simulink model "SCARA_Control_System"  (R2023a)
settings: Solver=VariableStepAuto  StartTime=0.0  StopTime=10.0  RelTol=1e-3
undefined symbols (not defined in the file): X, Y, Z
libraries: sm_lib x25, nesl_utility x16, robotcorelib x1
settings Model: Creator=Memoh  LastModifiedBy=Memoh

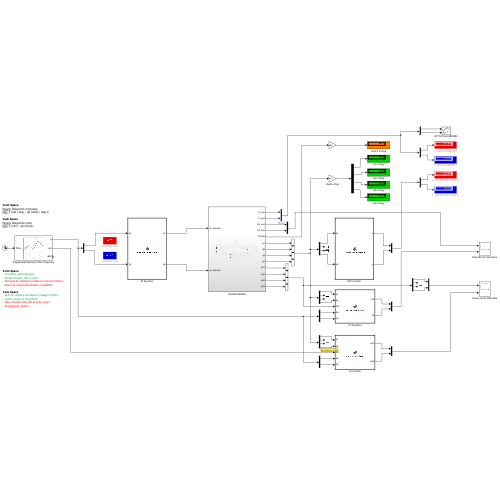
[thumbnail: Simulink's stored preview of the top-level diagram]
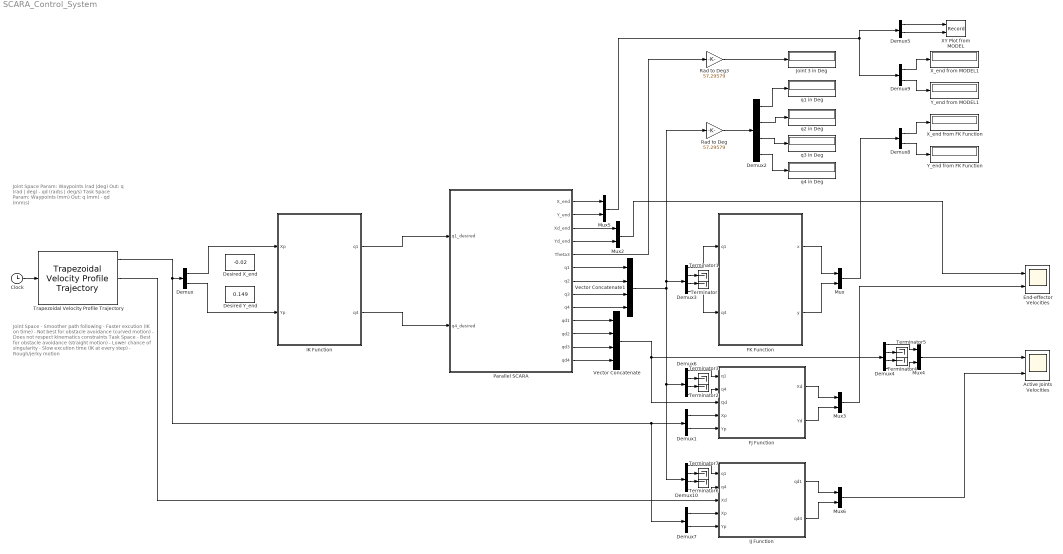
== system SCARA_Control_System ==
  note: Joint Space
      | Param: Waypoints (rad |deg)
      | Out: q (rad | deg) - qd (rad\s | deg/s)
      |
      | Task Space
      | Param: Waypoints (mm)
      | Out: q (mm) - qd (mm\s)
  note: Joint Space
      | - Smoother path following
      | - Faster excution (IK on time)
      | - Not best for obstacle avoidance (curved motion)
      | - Does not respect kinematics constraints
      |
      | Task Space
      | - Best for obstacle avoidance (straight motion)
      | - Lower chance of singularity
      | - Slow excution time (IK at every step)
      | - Rough/jerky motion
  Active Joints Velocities : Scope  NumInputPorts=2
  Clock : Clock
  Demux{,1,5,7..9} (6 alike) : Demux  Outputs=2
  Demux{2..4,6,10} (5 alike) : Demux
  Desired X_end : Constant  Value=-0.02
  Desired Y_end : Constant  Value=0.149
  End-effector Velocities : Scope  NumInputPorts=2
  FJ Function : MATLAB Function  TreatAsAtomicUnit=on
  FK Function : MATLAB Function  TreatAsAtomicUnit=on
  IJ Function : MATLAB Function  TreatAsAtomicUnit=on
  IK Function : MATLAB Function  TreatAsAtomicUnit=on
  Joint 3 in Deg : Display
  Mux{,2..6} (6 alike) : Mux  Inputs=2
  Parallel SCARA : Subsystem
  Rad to Deg : Gain  Gain=57.29579
  Rad to Deg3 : Gain  Gain=57.29579
  Terminator{,1..7} (8 alike) : Terminator
  Trapezoidal Velocity Profile Trajectory : robotcorelib/Trapezoidal Velocity Profile Trajectory  WaypointSource=Internal  Waypoints=[-0.02 0.02 0.02 -0.02 -0.02; 0.15 0.15 0.25 0.25 0.149]  NumParams=1  Parameter1=End Time  Parameter2=End Time  ParameterSource=Internal  PeakVelocity=[ 10; 10]  Acceleration=5  EndTime=2  AccelTime=[ 1; 2 ]  SimulateUsing=Interpreted execution
  Vector Concatenate : Concatenate  NumInputs=4
  Vector Concatenate1 : Concatenate  NumInputs=4
  XY Plot from MODEL : Record  FileSettingsInternal="{\"entries\":[{\"content\":{\"excelSettings\":{\"content\":{},\"type\":\"Streamout.ExcelSettings\"}},\"type\":\"Streamout.FileSettingStorage\",\"uuid\":\"f4e9d8e9-783c-4af9-9f9e-7bd75a06b44d\"}],\"packageUris\":[\"http://schema.mathworks.com/mf0/streamout_blocks/R2020a\"],\"version\":\"1.0\"}"  Layout=[1 1]  SignalsInternal="{\"entries\":[{\"content\":{\"signals\":[{\"content\":{\"blockPath\":[\"SCARA_Control_System/XY Plot from MODEL\"],\"dimensions\":[1],\"domain\":\"SCARA_Control_System/XY Plot from MODEL\",\"lineColor\":\"#22b573\",\"port\":1,\"sid\":[\"\"],\"signalID\":1875,\"signalName\":\"Demux5:1\"},\"type\":\"RecordBlkView.Signal\",\"uuid\":\"6f077d22-c755-4374-a6e7-1c1d86a9b0c2\"},{\"content\":{\"blockPath\":[\"SCARA_Control_System/XY Plot from MODEL\"],\"dimensions\":[1],\"domain\":\"SCARA_Control_System/XY Plot from MODEL\",\"lineColor\":\"#0072bd\",\"port\":2,\"sid\":[\"\"],\"signalID\":1879,\"signalName\":\"Demux5:2\"},\"type\":\"RecordBlkView.Signal\",\"uuid\":\"b8998448-4b25-43e1-97c9-c4fbc39d53c5\"}]},\"type\":\"RecordBlkView.InputSignals\",\"uuid\":\"f1e410ec-52b3-42c9-84f2-8d8e914f3791\"}],\"packageUris\":[\"http://schema.mathworks.com/mf0/streamout_blocks/R2020a\"],\"version\":\"1.0\"}"  VisualizationBindings="{\"xyplotplugin\":{\"info\":[{\"series\":[],\"subplotID\":1}]}}"  CompatibilityTag=XY
  X_end from FK Function : Display
  X_end from MODEL1 : Display
  Y_end from FK Function : Display
  Y_end from MODEL1 : Display
  q1 in Deg : Display
  q2 in Deg : Display
  q3 in Deg : Display
  q4 in Deg : Display
  wires:
  Parallel SCARA/6(q1) -> Vector Concatenate1/1
  FK Function/1(x) -> Mux/1
  FK Function/2(y) -> Mux/2
  Clock/1 -> Trapezoidal Velocity Profile Trajectory/1
  Trapezoidal Velocity Profile Trajectory/1 -> Demux7/1, Demux1/1, Demux/1
  Parallel SCARA/10(qd1) -> Vector Concatenate/1
  Parallel SCARA/11(qd2) -> Vector Concatenate/2
  Parallel SCARA/12(qd3) -> Vector Concatenate/3
  Parallel SCARA/13(qd4) -> Vector Concatenate/4
  Parallel SCARA/3(Xd_end) -> Mux2/1
  Parallel SCARA/4(Yd_end) -> Mux2/2
  Rad to Deg/1 -> Demux2/1
  Demux2/1 -> q1 in Deg/1
  Demux2/2 -> q2 in Deg/1
  Demux2/3 -> q3 in Deg/1
  Demux2/4 -> q4 in Deg/1
  FJ Function/2(Yd) -> Mux3/2
  FJ Function/1(Xd) -> Mux3/1
  Parallel SCARA/7(q2) -> Vector Concatenate1/2
  Parallel SCARA/8(q3) -> Vector Concatenate1/3
  Rad to Deg3/1 -> Joint 3 in Deg/1
  Parallel SCARA/5(Theta3) -> Rad to Deg3/1
  Mux3/1 -> End-effector Velocities/2
  Demux/1 -> IK Function/1(Xp)
  Demux/2 -> IK Function/2(Yp)
  IK Function/1(q1) -> Parallel SCARA/1(q1_desired)
  IK Function/2(q4) -> Parallel SCARA/2(q4_desired)
  Demux3/3 -> Terminator/1
  Demux3/2 -> Terminator1/1
  Demux3/1 -> FK Function/1(q1)
  Demux3/4 -> FK Function/2(q4)
  Parallel SCARA/9(q4) -> Vector Concatenate1/4
  Parallel SCARA/1(X_end) -> Mux5/1
  Parallel SCARA/2(Y_end) -> Mux5/2
  Demux5/1 -> XY Plot from MODEL/1
  Demux5/2 -> XY Plot from MODEL/2
  Demux6/3 -> Terminator2/1
  Demux6/2 -> Terminator3/1
  Demux6/1 -> FJ Function/1(q1)
  Demux6/4 -> FJ Function/2(q4)
  Demux1/2 -> FJ Function/5(Yp)
  Trapezoidal Velocity Profile Trajectory/2 -> IJ Function/3(Xd)
  Demux8/2 -> Y_end from FK Function/1
  Demux8/1 -> X_end from FK Function/1
  Mux/1 -> Demux8/1
  Demux9/2 -> Y_end from MODEL1/1
  Demux9/1 -> X_end from MODEL1/1
  Mux5/1 -> Demux9/1, Demux5/1
  Mux2/1 -> End-effector Velocities/1
  Demux4/3 -> Terminator4/1
  Demux4/2 -> Terminator5/1
  Demux4/4 -> Mux4/2
  Demux4/1 -> Mux4/1
  Mux4/1 -> Active Joints Velocities/1
  IJ Function/1(qd1) -> Mux6/1
  IJ Function/2(qd4) -> Mux6/2
  Mux6/1 -> Active Joints Velocities/2
  Demux7/1 -> IJ Function/4(Xp)
  Demux10/3 -> Terminator6/1
  Demux7/2 -> IJ Function/5(Yp)
  Demux10/2 -> Terminator7/1
  Vector Concatenate1/1 -> Rad to Deg/1, Demux3/1, Demux10/1, Demux6/1
  Demux10/4 -> IJ Function/2(q4)
  Demux10/1 -> IJ Function/1(q1)
  Demux1/1 -> FJ Function/4(Xp)
  Vector Concatenate/1 -> FJ Function/3(Qd), Demux4/1

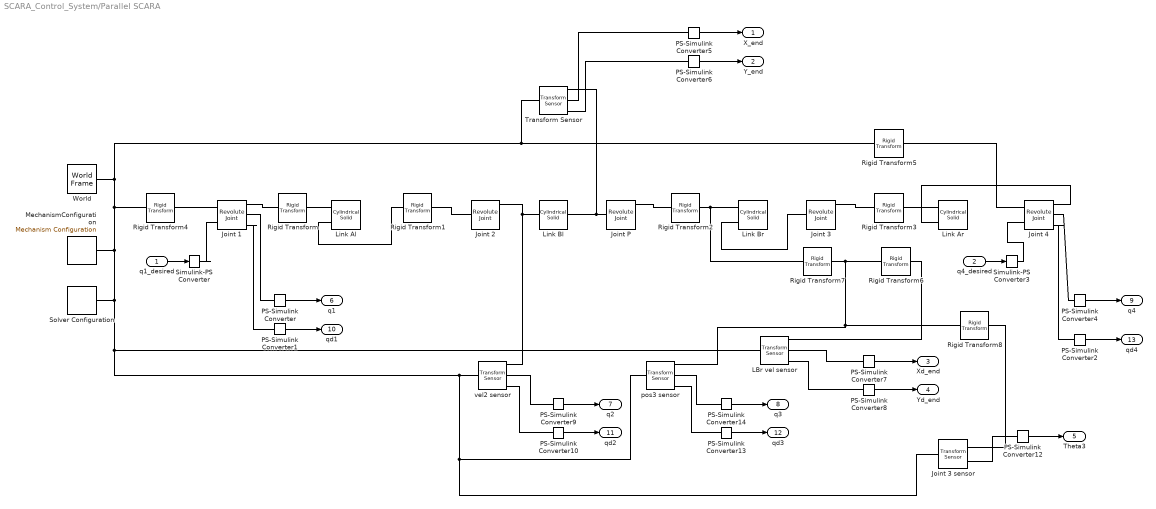
== system SCARA_Control_System/Parallel SCARA ==
  q1_desired : Inport
  q4_desired : Inport  Port=2
  Joint 1 : sm_lib/Joints/Revolute Joint  JointMode=Normal  SenseConstraintForce=off  SenseConstraintForceX=off  SenseConstraintForceY=off  SenseConstraintForceZ=off  SenseConstraintTorque=off  SenseConstraintTorqueX=off  SenseConstraintTorqueY=off  SenseConstraintTorqueZ=off  SenseTotalForce=off  SenseTotalForceX=off  SenseTotalForceY=off  SenseTotalForceZ=off  SenseTotalTorque=off  SenseTotalTorqueX=off  SenseTotalTorqueY=off  SenseTotalTorqueZ=off  CompositeWrenchDir=FollowerOnBase  CompositeWrenchFrame=BaseFrame  EquilibriumPosition=0  EquilibriumPositionUnits=deg  SpringStiffness=0  SpringStiffnessUnits=N*m/deg  DampingCoefficient=0  DampingCoefficientUnits=N*m/(deg/s)  TorqueActuationMode=ComputedTorque  MotionActuationMode=InputMotion  SensePosition=on  SenseVelocity=on  SenseAcceleration=off  SenseTorqueForce=off  SenseLowerLimitTorqueForce=off  SenseUpperLimitTorqueForce=off  LowerLimitSpecify=off  LowerLimitBound=-90  LowerLimitBoundUnits=deg  LowerLimitStiffness=1e4  LowerLimitStiffnessUnits=N*m/deg  LowerLimitDamping=10  LowerLimitDampingUnits=N*m/(deg/s)  LowerLimitTransitionRegionWidth=0.1  LowerLimitTransitionRegionWidthUnits=deg  UpperLimitSpecify=off  UpperLimitBound=90  UpperLimitBoundUnits=deg  UpperLimitStiffness=1e4  UpperLimitStiffnessUnits=N*m/deg  UpperLimitDamping=10  UpperLimitDampingUnits=N*m/(deg/s)  UpperLimitTransitionRegionWidth=0.1  UpperLimitTransitionRegionWidthUnits=deg  PositionTargetSpecify=on  PositionTargetPriority=High  PositionTargetValue=90  PositionTargetValueUnits=deg  VelocityTargetSpecify=off  VelocityTargetPriority=High  VelocityTargetValue=0  VelocityTargetValueUnits=deg/s
  Joint 2 : sm_lib/Joints/Revolute Joint  JointMode=Normal  SenseConstraintForce=off  SenseConstraintForceX=off  SenseConstraintForceY=off  SenseConstraintForceZ=off  SenseConstraintTorque=off  SenseConstraintTorqueX=off  SenseConstraintTorqueY=off  SenseConstraintTorqueZ=off  SenseTotalForce=off  SenseTotalForceX=off  SenseTotalForceY=off  SenseTotalForceZ=off  SenseTotalTorque=off  SenseTotalTorqueX=off  SenseTotalTorqueY=off  SenseTotalTorqueZ=off  CompositeWrenchDir=FollowerOnBase  CompositeWrenchFrame=BaseFrame  EquilibriumPosition=0  EquilibriumPositionUnits=deg  SpringStiffness=0  SpringStiffnessUnits=N*m/deg  DampingCoefficient=0  DampingCoefficientUnits=N*m/(deg/s)  TorqueActuationMode=NoTorque  MotionActuationMode=ComputedMotion  SensePosition=on  SenseVelocity=on  SenseAcceleration=off  SenseTorqueForce=off  SenseLowerLimitTorqueForce=off  SenseUpperLimitTorqueForce=off  LowerLimitSpecify=off  LowerLimitBound=-90  LowerLimitBoundUnits=deg  LowerLimitStiffness=1e4  LowerLimitStiffnessUnits=N*m/deg  LowerLimitDamping=10  LowerLimitDampingUnits=N*m/(deg/s)  LowerLimitTransitionRegionWidth=0.1  LowerLimitTransitionRegionWidthUnits=deg  UpperLimitSpecify=off  UpperLimitBound=90  UpperLimitBoundUnits=deg  UpperLimitStiffness=1e4  UpperLimitStiffnessUnits=N*m/deg  UpperLimitDamping=10  UpperLimitDampingUnits=N*m/(deg/s)  UpperLimitTransitionRegionWidth=0.1  UpperLimitTransitionRegionWidthUnits=deg  PositionTargetSpecify=on  PositionTargetPriority=Low  PositionTargetValue=0  PositionTargetValueUnits=deg  VelocityTargetSpecify=off  VelocityTargetPriority=High  VelocityTargetValue=0  VelocityTargetValueUnits=deg/s
  Joint 3 : sm_lib/Joints/Revolute Joint  JointMode=Normal  SenseConstraintForce=off  SenseConstraintForceX=off  SenseConstraintForceY=off  SenseConstraintForceZ=off  SenseConstraintTorque=off  SenseConstraintTorqueX=off  SenseConstraintTorqueY=off  SenseConstraintTorqueZ=off  SenseTotalForce=off  SenseTotalForceX=off  SenseTotalForceY=off  SenseTotalForceZ=off  SenseTotalTorque=off  SenseTotalTorqueX=off  SenseTotalTorqueY=off  SenseTotalTorqueZ=off  CompositeWrenchDir=FollowerOnBase  CompositeWrenchFrame=BaseFrame  EquilibriumPosition=0  EquilibriumPositionUnits=deg  SpringStiffness=0  SpringStiffnessUnits=N*m/deg  DampingCoefficient=0  DampingCoefficientUnits=N*m/(deg/s)  TorqueActuationMode=NoTorque  MotionActuationMode=ComputedMotion  SensePosition=on  SenseVelocity=on  SenseAcceleration=off  SenseTorqueForce=off  SenseLowerLimitTorqueForce=off  SenseUpperLimitTorqueForce=off  LowerLimitSpecify=off  LowerLimitBound=-90  LowerLimitBoundUnits=deg  LowerLimitStiffness=1e4  LowerLimitStiffnessUnits=N*m/deg  LowerLimitDamping=10  LowerLimitDampingUnits=N*m/(deg/s)  LowerLimitTransitionRegionWidth=0.1  LowerLimitTransitionRegionWidthUnits=deg  UpperLimitSpecify=off  UpperLimitBound=90  UpperLimitBoundUnits=deg  UpperLimitStiffness=1e4  UpperLimitStiffnessUnits=N*m/deg  UpperLimitDamping=10  UpperLimitDampingUnits=N*m/(deg/s)  UpperLimitTransitionRegionWidth=0.1  UpperLimitTransitionRegionWidthUnits=deg  PositionTargetSpecify=off  PositionTargetPriority=High  PositionTargetValue=0  PositionTargetValueUnits=deg  VelocityTargetSpecify=off  VelocityTargetPriority=High  VelocityTargetValue=0  VelocityTargetValueUnits=deg/s
  "Joint 3 sensor " : sm_lib/Frames and Transforms/Transform Sensor  MeasurementFrame=Base  RotationSequence=YXY  SenseAngle=on  SenseAxis=off  SenseQ=off  SenseR=off  SenseRotationSequence=off  SenseOmegaX=off  SenseOmegaY=off  SenseOmegaZ=off  SenseQDot=off  SenseRDot=off  SenseRotationSequenceDot=off  SenseAlphaX=off  SenseAlphaY=off  SenseAlphaZ=off  SenseQDDot=off  SenseRDDot=off  SenseX=off  SenseY=off  SenseZ=off  SenseRad=off  SenseAzim=off  SenseDist=off  SenseInc=off  SenseXDot=off  SenseYDot=off  SenseZDot=off  SenseRadDot=off  SenseAzimDot=off  SenseDistDot=off  SenseIncDot=off  SenseXDDot=off  SenseYDDot=off  SenseZDDot=off  SenseRadDDot=off  SenseAzimDDot=off  SenseDistDDot=off  SenseIncDDot=off
  Joint 4 : sm_lib/Joints/Revolute Joint  JointMode=Normal  SenseConstraintForce=off  SenseConstraintForceX=off  SenseConstraintForceY=off  SenseConstraintForceZ=off  SenseConstraintTorque=off  SenseConstraintTorqueX=off  SenseConstraintTorqueY=off  SenseConstraintTorqueZ=off  SenseTotalForce=off  SenseTotalForceX=off  SenseTotalForceY=off  SenseTotalForceZ=off  SenseTotalTorque=off  SenseTotalTorqueX=off  SenseTotalTorqueY=off  SenseTotalTorqueZ=off  CompositeWrenchDir=FollowerOnBase  CompositeWrenchFrame=BaseFrame  EquilibriumPosition=0  EquilibriumPositionUnits=deg  SpringStiffness=0  SpringStiffnessUnits=N*m/deg  DampingCoefficient=0  DampingCoefficientUnits=N*m/(deg/s)  TorqueActuationMode=ComputedTorque  MotionActuationMode=InputMotion  SensePosition=on  SenseVelocity=on  SenseAcceleration=off  SenseTorqueForce=off  SenseLowerLimitTorqueForce=off  SenseUpperLimitTorqueForce=off  LowerLimitSpecify=off  LowerLimitBound=-90  LowerLimitBoundUnits=deg  LowerLimitStiffness=1e4  LowerLimitStiffnessUnits=N*m/deg  LowerLimitDamping=10  LowerLimitDampingUnits=N*m/(deg/s)  LowerLimitTransitionRegionWidth=0.1  LowerLimitTransitionRegionWidthUnits=deg  UpperLimitSpecify=off  UpperLimitBound=90  UpperLimitBoundUnits=deg  UpperLimitStiffness=1e4  UpperLimitStiffnessUnits=N*m/deg  UpperLimitDamping=10  UpperLimitDampingUnits=N*m/(deg/s)  UpperLimitTransitionRegionWidth=0.1  UpperLimitTransitionRegionWidthUnits=deg  PositionTargetSpecify=on  PositionTargetPriority=High  PositionTargetValue=90  PositionTargetValueUnits=deg  VelocityTargetSpecify=off  VelocityTargetPriority=High  VelocityTargetValue=0  VelocityTargetValueUnits=deg/s
  Joint P : sm_lib/Joints/Revolute Joint  JointMode=Normal  SenseConstraintForce=off  SenseConstraintForceX=off  SenseConstraintForceY=off  SenseConstraintForceZ=off  SenseConstraintTorque=off  SenseConstraintTorqueX=off  SenseConstraintTorqueY=off  SenseConstraintTorqueZ=off  SenseTotalForce=off  SenseTotalForceX=off  SenseTotalForceY=off  SenseTotalForceZ=off  SenseTotalTorque=off  SenseTotalTorqueX=off  SenseTotalTorqueY=off  SenseTotalTorqueZ=off  CompositeWrenchDir=FollowerOnBase  CompositeWrenchFrame=BaseFrame  EquilibriumPosition=0  EquilibriumPositionUnits=deg  SpringStiffness=0  SpringStiffnessUnits=N*m/deg  DampingCoefficient=0  DampingCoefficientUnits=N*m/(deg/s)  TorqueActuationMode=NoTorque  MotionActuationMode=ComputedMotion  SensePosition=on  SenseVelocity=on  SenseAcceleration=off  SenseTorqueForce=off  SenseLowerLimitTorqueForce=off  SenseUpperLimitTorqueForce=off  LowerLimitSpecify=off  LowerLimitBound=-90  LowerLimitBoundUnits=deg  LowerLimitStiffness=1e4  LowerLimitStiffnessUnits=N*m/deg  LowerLimitDamping=10  LowerLimitDampingUnits=N*m/(deg/s)  LowerLimitTransitionRegionWidth=0.1  LowerLimitTransitionRegionWidthUnits=deg  UpperLimitSpecify=off  UpperLimitBound=90  UpperLimitBoundUnits=deg  UpperLimitStiffness=1e4  UpperLimitStiffnessUnits=N*m/deg  UpperLimitDamping=10  UpperLimitDampingUnits=N*m/(deg/s)  UpperLimitTransitionRegionWidth=0.1  UpperLimitTransitionRegionWidthUnits=deg  PositionTargetSpecify=off  PositionTargetPriority=High  PositionTargetValue=0  PositionTargetValueUnits=deg  VelocityTargetSpecify=off  VelocityTargetPriority=High  VelocityTargetValue=0  VelocityTargetValueUnits=deg/s
  LBr vel sensor : sm_lib/Frames and Transforms/Transform Sensor  MeasurementFrame=Base  RotationSequence=YXY  SenseAngle=off  SenseAxis=off  SenseQ=off  SenseR=off  SenseRotationSequence=off  SenseOmegaX=off  SenseOmegaY=off  SenseOmegaZ=off  SenseQDot=off  SenseRDot=off  SenseRotationSequenceDot=off  SenseAlphaX=off  SenseAlphaY=off  SenseAlphaZ=off  SenseQDDot=off  SenseRDDot=off  SenseX=off  SenseY=off  SenseZ=off  SenseRad=off  SenseAzim=off  SenseDist=off  SenseInc=off  SenseXDot=on  SenseYDot=on  SenseZDot=off  SenseRadDot=off  SenseAzimDot=off  SenseDistDot=off  SenseIncDot=off  SenseXDDot=off  SenseYDDot=off  SenseZDDot=off  SenseRadDDot=off  SenseAzimDDot=off  SenseDistDDot=off  SenseIncDDot=off
  Link Al : sm_lib/Body Elements/Cylindrical Solid  GraphicAmbientColor=[0.15 0.15 0.15 1.0]  BasedOnType=Density  CenterOfMass=[0 0 0]  CenterOfMassUnits=m  GraphicDiffuseColor=[1.0 0.0 0.0]  CylinderLength=0.100  CylinderLengthUnits=m  CylinderRadius=0.010  CylinderRadiusUnits=m  Density=1000  DensityUnits=kg/m^3  DoExposeReferenceFrame=on  GraphicEmissiveColor=[0.0 0.0 0.0 1.0]  ExportEntireGeometry=off  SerializedFrames=<Frames><Frame><Id>Frame1</Id><Value><Name>F1</Name><Origin><Source>GeometricFeature</Source><FeatureName>bottom surface</FeatureName></Origin><PrimaryAxis><DefinedDirection>+Y</DefinedDirection><Source>ReferenceFrame</Source><SourceDirection>+Y</SourceDirection><FeatureName></FeatureName></PrimaryAxis><SecondaryAxis><DefinedDirection>+X</DefinedDirection><Source>ReferenceFrame</Source><SourceDirection>+X</SourceDirection><FeatureName></FeatureName></SecondaryAxis></Value></Frame><Frame><Id>Frame2</Id><Value><Name>F2</Name><Origin><Source>GeometricFeature</Source><FeatureName>top surface</FeatureName></Origin><PrimaryAxis><DefinedDirection>+Z</DefinedDirection><Source>ReferenceFrame</Source><SourceDirection>+Z</SourceDirection><FeatureName></FeatureName></PrimaryAxis><SecondaryAxis><DefinedDirection>+X</DefinedDirection><Source>ReferenceFrame</Source><SourceDirection>+X</SourceDirection><FeatureName></FeatureName></SecondaryAxis></Value></Frame></Frames>  MarkerShape=Sphere  MarkerSize=10  GraphicType=FromGeometry  InertiaType=CalculateFromGeometry  Mass=1  MassUnits=kg  MomentsOfInertia=[1 1 1]  MomentsOfInertiaUnits=kg*m^2  GraphicOpacity=1.0  ProductsOfInertia=[0 0 0]  ProductsOfInertiaUnits=kg*m^2  GraphicShininess=75  GraphicSpecularColor=[0.5 0.5 0.5 1.0]  GraphicVisPropType=SimpleVisualProperties
  Link Ar : sm_lib/Body Elements/Cylindrical Solid  GraphicAmbientColor=[0.15 0.15 0.15 1.0]  BasedOnType=Density  CenterOfMass=[0 0 0]  CenterOfMassUnits=m  GraphicDiffuseColor=[0.2 0.0 0.8]  CylinderLength=0.100  CylinderLengthUnits=m  CylinderRadius=0.01  CylinderRadiusUnits=m  Density=1000  DensityUnits=kg/m^3  DoExposeReferenceFrame=on  GraphicEmissiveColor=[0.0 0.0 0.0 1.0]  ExportEntireGeometry=off  SerializedFrames=<Frames><Frame><Id>Frame1</Id><Value><Name>F1</Name><Origin><Source>GeometricFeature</Source><FeatureName>bottom surface</FeatureName></Origin><PrimaryAxis><DefinedDirection>+Z</DefinedDirection><Source>ReferenceFrame</Source><SourceDirection>+Z</SourceDirection><FeatureName></FeatureName></PrimaryAxis><SecondaryAxis><DefinedDirection>+X</DefinedDirection><Source>ReferenceFrame</Source><SourceDirection>+X</SourceDirection><FeatureName></FeatureName></SecondaryAxis></Value></Frame><Frame><Id>Frame2</Id><Value><Name>F2</Name><Origin><Source>GeometricFeature</Source><FeatureName>top surface</FeatureName></Origin><PrimaryAxis><DefinedDirection>+X</DefinedDirection><Source>ReferenceFrame</Source><SourceDirection>-Z</SourceDirection><FeatureName></FeatureName></PrimaryAxis><SecondaryAxis><DefinedDirection>+Y</DefinedDirection><Source>ReferenceFrame</Source><SourceDirection>+Y</SourceDirection><FeatureName></FeatureName></SecondaryAxis></Value></Frame></Frames>  MarkerShape=Sphere  MarkerSize=10  GraphicType=FromGeometry  InertiaType=CalculateFromGeometry  Mass=1  MassUnits=kg  MomentsOfInertia=[1 1 1]  MomentsOfInertiaUnits=kg*m^2  GraphicOpacity=1.0  ProductsOfInertia=[0 0 0]  ProductsOfInertiaUnits=kg*m^2  GraphicShininess=75  GraphicSpecularColor=[0.5 0.5 0.5 1.0]  GraphicVisPropType=SimpleVisualProperties
  Link Bl : sm_lib/Body Elements/Cylindrical Solid  GraphicAmbientColor=[0.15 0.15 0.15 1.0]  BasedOnType=Density  CenterOfMass=[0 0 0]  CenterOfMassUnits=m  GraphicDiffuseColor=[1.0 0.6 0.0]  CylinderLength=0.220  CylinderLengthUnits=m  CylinderRadius=0.01  CylinderRadiusUnits=m  Density=1000  DensityUnits=kg/m^3  DoExposeReferenceFrame=off  GraphicEmissiveColor=[0.0 0.0 0.0 1.0]  ExportEntireGeometry=off  SerializedFrames=<Frames><Frame><Id>Frame1</Id><Value><Name>F1</Name><Origin><Source>GeometricFeature</Source><FeatureName>bottom surface</FeatureName></Origin><PrimaryAxis><DefinedDirection>+Z</DefinedDirection><Source>ReferenceFrame</Source><SourceDirection>-X</SourceDirection><FeatureName></FeatureName></PrimaryAxis><SecondaryAxis><DefinedDirection>+X</DefinedDirection><Source>ReferenceFrame</Source><SourceDirection>+Z</SourceDirection><FeatureName></FeatureName></SecondaryAxis></Value></Frame><Frame><Id>Frame2</Id><Value><Name>F2</Name><Origin><Source>GeometricFeature</Source><FeatureName>top surface</FeatureName></Origin><PrimaryAxis><DefinedDirection>+X</DefinedDirection><Source>ReferenceFrame</Source><SourceDirection>+Z</SourceDirection><FeatureName></FeatureName></PrimaryAxis><SecondaryAxis><DefinedDirection>+Z</DefinedDirection><Source>ReferenceFrame</Source><SourceDirection>-X</SourceDirection><FeatureName></FeatureName></SecondaryAxis></Value></Frame></Frames>  MarkerShape=Sphere  MarkerSize=10  GraphicType=FromGeometry  InertiaType=CalculateFromGeometry  Mass=1  MassUnits=kg  MomentsOfInertia=[1 1 1]  MomentsOfInertiaUnits=kg*m^2  GraphicOpacity=1.0  ProductsOfInertia=[0 0 0]  ProductsOfInertiaUnits=kg*m^2  GraphicShininess=75  GraphicSpecularColor=[0.5 0.5 0.5 1.0]  GraphicVisPropType=SimpleVisualProperties
  Link Br : sm_lib/Body Elements/Cylindrical Solid  GraphicAmbientColor=[0.15 0.15 0.15 1.0]  BasedOnType=Density  CenterOfMass=[0 0 0]  CenterOfMassUnits=m  GraphicDiffuseColor=[0.6 1.0 0.0]  CylinderLength=0.220  CylinderLengthUnits=m  CylinderRadius=0.01  CylinderRadiusUnits=m  Density=1000  DensityUnits=kg/m^3  DoExposeReferenceFrame=on  GraphicEmissiveColor=[0.0 0.0 0.0 1.0]  ExportEntireGeometry=off  SerializedFrames=<Frames><Frame><Id>Frame1</Id><Value><Name>F1</Name><Origin><Source>GeometricFeature</Source><FeatureName>bottom surface</FeatureName></Origin><PrimaryAxis><DefinedDirection>+Z</DefinedDirection><Source>ReferenceFrame</Source><SourceDirection>+Z</SourceDirection><FeatureName></FeatureName></PrimaryAxis><SecondaryAxis><DefinedDirection>+X</DefinedDirection><Source>ReferenceFrame</Source><SourceDirection>+X</SourceDirection><FeatureName></FeatureName></SecondaryAxis></Value></Frame><Frame><Id>Frame2</Id><Value><Name>F2</Name><Origin><Source>GeometricFeature</Source><FeatureName>top surface</FeatureName></Origin><PrimaryAxis><DefinedDirection>+Y</DefinedDirection><Source>ReferenceFrame</Source><SourceDirection>-Z</SourceDirection><FeatureName></FeatureName></PrimaryAxis><SecondaryAxis><DefinedDirection>+Z</DefinedDirection><Source>ReferenceFrame</Source><SourceDirection>+Y</SourceDirection><FeatureName></FeatureName></SecondaryAxis></Value></Frame></Frames>  MarkerShape=Sphere  MarkerSize=10  GraphicType=FromGeometry  InertiaType=CalculateFromGeometry  Mass=1  MassUnits=kg  MomentsOfInertia=[1 1 1]  MomentsOfInertiaUnits=kg*m^2  GraphicOpacity=1.0  ProductsOfInertia=[0 0 0]  ProductsOfInertiaUnits=kg*m^2  GraphicShininess=75  GraphicSpecularColor=[0.5 0.5 0.5 1.0]  GraphicVisPropType=SimpleVisualProperties
  MechanismConfiguration : sm_lib/Utilities/Mechanism Configuration  UniformGravity=Constant  GravityVector=[0 0 -9.80665]  GravityVectorUnits=m/s^2  LinearizationDelta=0.001  JointModeTransitionNonlinearIterations=2
  PS-Simulink Converter{,1..2,4..10,12..14} (13 alike) : nesl_utility/PS-Simulink Converter  PhysicalDomain=network_engine_domain  SubClassName=ps_output  LeftPortType=input  RightPortType=output  PseudoPeriodic=off  Frequencies=[]  VectorFormat=inherit  Unit=inherit  AffineConversion=off
  Rigid Transform : sm_lib/Frames and Transforms/Rigid Transform  TranslationMethod=None  TranslationStandardOffset=0  TranslationStandardOffsetUnits=m  TranslationStandardAxis=+Z  TranslationCartesianOffset=[0 0 0]  TranslationCartesianOffsetUnits=m  TranslationROffset=0  TranslationROffsetUnits=m  TranslationZOffset=0  TranslationZOffsetUnits=m  TranslationThetaOffset=0  TranslationThetaOffsetUnits=deg  RotationMethod=StandardAxis  RotationAngleUnits=deg  RotationStandardAxis=-X  RotationAngle=90  RotationArbitraryAxis=[0 0 1]  FollAlignAxisA=+X  BaseAlignAxisA=+Y  FollAlignAxisB=+Y  BaseAlignAxisB=+Z  RotationSequenceAxes=FollowerAxes  RotationSequence=XYX  RotationSequenceAngles=[0 0 0]  RotationSequenceAnglesUnits=deg  RotationMatrix=[1 0 0; 0 1 0; 0 0 1]  Quaternion=[1 0 0 0]
  Rigid Transform1 : sm_lib/Frames and Transforms/Rigid Transform  TranslationMethod=None  TranslationStandardOffset=0  TranslationStandardOffsetUnits=m  TranslationStandardAxis=+Z  TranslationCartesianOffset=[0 0 0]  TranslationCartesianOffsetUnits=m  TranslationROffset=0  TranslationROffsetUnits=m  TranslationZOffset=0  TranslationZOffsetUnits=m  TranslationThetaOffset=0  TranslationThetaOffsetUnits=deg  RotationMethod=StandardAxis  RotationAngleUnits=deg  RotationStandardAxis=+X  RotationAngle=90  RotationArbitraryAxis=[0 0 1]  FollAlignAxisA=+X  BaseAlignAxisA=+Y  FollAlignAxisB=+Y  BaseAlignAxisB=+Z  RotationSequenceAxes=FollowerAxes  RotationSequence=XYX  RotationSequenceAngles=[0 0 0]  RotationSequenceAnglesUnits=deg  RotationMatrix=[1 0 0; 0 1 0; 0 0 1]  Quaternion=[1 0 0 0]
  Rigid Transform2 : sm_lib/Frames and Transforms/Rigid Transform  TranslationMethod=None  TranslationStandardOffset=0  TranslationStandardOffsetUnits=m  TranslationStandardAxis=+Z  TranslationCartesianOffset=[0 0 0]  TranslationCartesianOffsetUnits=m  TranslationROffset=0  TranslationROffsetUnits=m  TranslationZOffset=0  TranslationZOffsetUnits=m  TranslationThetaOffset=0  TranslationThetaOffsetUnits=deg  RotationMethod=StandardAxis  RotationAngleUnits=deg  RotationStandardAxis=+X  RotationAngle=90  RotationArbitraryAxis=[0 0 1]  FollAlignAxisA=+X  BaseAlignAxisA=+Y  FollAlignAxisB=+Y  BaseAlignAxisB=+Z  RotationSequenceAxes=FollowerAxes  RotationSequence=XYX  RotationSequenceAngles=[0 0 0]  RotationSequenceAnglesUnits=deg  RotationMatrix=[1 0 0; 0 1 0; 0 0 1]  Quaternion=[1 0 0 0]
  Rigid Transform3 : sm_lib/Frames and Transforms/Rigid Transform  TranslationMethod=None  TranslationStandardOffset=0  TranslationStandardOffsetUnits=m  TranslationStandardAxis=+Z  TranslationCartesianOffset=[0 0 0]  TranslationCartesianOffsetUnits=m  TranslationROffset=0  TranslationROffsetUnits=m  TranslationZOffset=0  TranslationZOffsetUnits=m  TranslationThetaOffset=0  TranslationThetaOffsetUnits=deg  RotationMethod=StandardAxis  RotationAngleUnits=deg  RotationStandardAxis=-Y  RotationAngle=90  RotationArbitraryAxis=[0 0 1]  FollAlignAxisA=+X  BaseAlignAxisA=+Y  FollAlignAxisB=+Y  BaseAlignAxisB=+Z  RotationSequenceAxes=FollowerAxes  RotationSequence=XYX  RotationSequenceAngles=[0 0 0]  RotationSequenceAnglesUnits=deg  RotationMatrix=[1 0 0; 0 1 0; 0 0 1]  Quaternion=[1 0 0 0]
  Rigid Transform4 : sm_lib/Frames and Transforms/Rigid Transform  TranslationMethod=Cartesian  TranslationStandardOffset=0  TranslationStandardOffsetUnits=m  TranslationStandardAxis=+Z  TranslationCartesianOffset=[-0.115 0 0]  TranslationCartesianOffsetUnits=m  TranslationROffset=0  TranslationROffsetUnits=m  TranslationZOffset=0  TranslationZOffsetUnits=m  TranslationThetaOffset=0  TranslationThetaOffsetUnits=deg  RotationMethod=StandardAxis  RotationAngleUnits=deg  RotationStandardAxis=-Z  RotationAngle=90  RotationArbitraryAxis=[0 0 1]  FollAlignAxisA=+X  BaseAlignAxisA=+Y  FollAlignAxisB=+Y  BaseAlignAxisB=+Z  RotationSequenceAxes=FollowerAxes  RotationSequence=XYX  RotationSequenceAngles=[0 0 0]  RotationSequenceAnglesUnits=deg  RotationMatrix=[1 0 0; 0 1 0; 0 0 1]  Quaternion=[1 0 0 0]
  Rigid Transform5 : sm_lib/Frames and Transforms/Rigid Transform  TranslationMethod=Cartesian  TranslationStandardOffset=0  TranslationStandardOffsetUnits=m  TranslationStandardAxis=+Z  TranslationCartesianOffset=[0.115 0 0]  TranslationCartesianOffsetUnits=m  TranslationROffset=0  TranslationROffsetUnits=m  TranslationZOffset=0  TranslationZOffsetUnits=m  TranslationThetaOffset=0  TranslationThetaOffsetUnits=deg  RotationMethod=None  RotationAngleUnits=deg  RotationStandardAxis=+Z  RotationAngle=0.0  RotationArbitraryAxis=[0 0 1]  FollAlignAxisA=+X  BaseAlignAxisA=+Y  FollAlignAxisB=+Y  BaseAlignAxisB=+Z  RotationSequenceAxes=FollowerAxes  RotationSequence=XYX  RotationSequenceAngles=[0 0 0]  RotationSequenceAnglesUnits=deg  RotationMatrix=[1 0 0; 0 1 0; 0 0 1]  Quaternion=[1 0 0 0]
  Rigid Transform6 : sm_lib/Frames and Transforms/Rigid Transform  TranslationMethod=Cartesian  TranslationStandardOffset=0  TranslationStandardOffsetUnits=m  TranslationStandardAxis=+Z  TranslationCartesianOffset=[0 0 0]  TranslationCartesianOffsetUnits=mm  TranslationROffset=0  TranslationROffsetUnits=m  TranslationZOffset=0  TranslationZOffsetUnits=m  TranslationThetaOffset=0  TranslationThetaOffsetUnits=deg  RotationMethod=None  RotationAngleUnits=deg  RotationStandardAxis=+Z  RotationAngle=90  RotationArbitraryAxis=[0 0 1]  FollAlignAxisA=+X  BaseAlignAxisA=+Y  FollAlignAxisB=+Y  BaseAlignAxisB=+Z  RotationSequenceAxes=FollowerAxes  RotationSequence=XYX  RotationSequenceAngles=[0 0 0]  RotationSequenceAnglesUnits=deg  RotationMatrix=[1 0 0; 0 1 0; 0 0 1]  Quaternion=[1 0 0 0]
  Rigid Transform7 : sm_lib/Frames and Transforms/Rigid Transform  TranslationMethod=None  TranslationStandardOffset=0  TranslationStandardOffsetUnits=m  TranslationStandardAxis=+Z  TranslationCartesianOffset=[0 0 0]  TranslationCartesianOffsetUnits=m  TranslationROffset=0  TranslationROffsetUnits=m  TranslationZOffset=0  TranslationZOffsetUnits=m  TranslationThetaOffset=0  TranslationThetaOffsetUnits=deg  RotationMethod=AlignedAxes  RotationAngleUnits=deg  RotationStandardAxis=+Z  RotationAngle=0.0  RotationArbitraryAxis=[0 0 1]  FollAlignAxisA=+Z  BaseAlignAxisA=+Y  FollAlignAxisB=+X  BaseAlignAxisB=+Z  RotationSequenceAxes=FollowerAxes  RotationSequence=XYX  RotationSequenceAngles=[0 0 0]  RotationSequenceAnglesUnits=deg  RotationMatrix=[1 0 0; 0 1 0; 0 0 1]  Quaternion=[1 0 0 0]
  Rigid Transform8 : sm_lib/Frames and Transforms/Rigid Transform  TranslationMethod=Cartesian  TranslationStandardOffset=0  TranslationStandardOffsetUnits=m  TranslationStandardAxis=+Z  TranslationCartesianOffset=[220 0 0]  TranslationCartesianOffsetUnits=mm  TranslationROffset=0  TranslationROffsetUnits=m  TranslationZOffset=0  TranslationZOffsetUnits=m  TranslationThetaOffset=0  TranslationThetaOffsetUnits=deg  RotationMethod=StandardAxis  RotationAngleUnits=deg  RotationStandardAxis=+Z  RotationAngle=180  RotationArbitraryAxis=[0 0 1]  FollAlignAxisA=+X  BaseAlignAxisA=+Y  FollAlignAxisB=+Y  BaseAlignAxisB=+Z  RotationSequenceAxes=FollowerAxes  RotationSequence=XYX  RotationSequenceAngles=[0 0 0]  RotationSequenceAnglesUnits=deg  RotationMatrix=[1 0 0; 0 1 0; 0 0 1]  Quaternion=[1 0 0 0]
  Simulink-PS Converter : nesl_utility/Simulink-PS Converter  PhysicalDomain=network_engine_domain  SubClassName=ps_input  LeftPortType=input  RightPortType=output  PseudoPeriodic=off  Frequencies=[]  NoiseDistribution=none  NoiseParameters=[]  Unit=1  AffineConversion=on  FilteringAndDerivatives=filter  SimscapeFilterOrder=2  InputFilterTimeConstant=0.001  UdotUserProvided=0
  Simulink-PS Converter3 : nesl_utility/Simulink-PS Converter  PhysicalDomain=network_engine_domain  SubClassName=ps_input  LeftPortType=input  RightPortType=output  PseudoPeriodic=off  Frequencies=[]  NoiseDistribution=none  NoiseParameters=[]  Unit=1  AffineConversion=on  FilteringAndDerivatives=filter  SimscapeFilterOrder=2  InputFilterTimeConstant=0.001  UdotUserProvided=0
  Solver Configuration : nesl_utility/Solver Configuration  PhysicalDomain=network_engine_domain  SubClassName=solver  LeftPortType=input  RightPortType=generic  Tones=[]  Harmonics=[]  SimulateNoise=off  Profile=off  UseLocalSampling=off  EnableSwitchedLinearOptims=on  FrequencyDomain=off  UseCCode=off  RelTol=0.001  AbsTol=0.001  MinStep=1e-09  ToWorkspace=off  RevertToSquareIcSolve=off  NumHomotopyIterations=100  PhasorMode=off  PhasorModeNumHarmonics=1  ConsistencySolver=NEWTON_XTOL_AFTER_FTOL  IndexReductionMethod=DerivativeReplacement  DoDC=off  ResidualTolerance=1e-09  ConsistencyTolSource=GLOBAL  ConsistencyAbsTol=0.001  ConsistencyRelTol=0.001  ConsistencyTolFactor=0.001  UseLocalSolver=off  LocalSolverChoice=NE_BACKWARD_EULER_ADVANCER  ResolveIndetEquations=on  FunctionEvalNumThread=1  LocalSolverSampleTime=0.001  DoFixedCost=off  MaxNonlinIter=3  MaxModeIter=2  ComputeImpulses=off  ImpulseIterations=2  LinearAlgebra=auto  LinearAlgebraNumThread=0  EquationFormulation=NE_TIME_EF  DelaysMemoryBudget=1024  AutomaticFiltering=on  FilteringTimeConstant=0.001  PartitionStorageMethod=AS_NEEDED  PartitionMemoryBudget=1024  PartitionMethod=ROBUST
  Transform Sensor : sm_lib/Frames and Transforms/Transform Sensor  MeasurementFrame=World  RotationSequence=XYX  SenseAngle=off  SenseAxis=off  SenseQ=off  SenseR=off  SenseRotationSequence=off  SenseOmegaX=off  SenseOmegaY=off  SenseOmegaZ=off  SenseQDot=off  SenseRDot=off  SenseRotationSequenceDot=off  SenseAlphaX=off  SenseAlphaY=off  SenseAlphaZ=off  SenseQDDot=off  SenseRDDot=off  SenseX=on  SenseY=on  SenseZ=off  SenseRad=off  SenseAzim=off  SenseDist=off  SenseInc=off  SenseXDot=off  SenseYDot=off  SenseZDot=off  SenseRadDot=off  SenseAzimDot=off  SenseDistDot=off  SenseIncDot=off  SenseXDDot=off  SenseYDDot=off  SenseZDDot=off  SenseRadDDot=off  SenseAzimDDot=off  SenseDistDDot=off  SenseIncDDot=off
  World : sm_lib/Frames and Transforms/World Frame
  pos3 sensor : sm_lib/Frames and Transforms/Transform Sensor  MeasurementFrame=World  RotationSequence=XYX  SenseAngle=on  SenseAxis=off  SenseQ=off  SenseR=off  SenseRotationSequence=off  SenseOmegaX=off  SenseOmegaY=off  SenseOmegaZ=on  SenseQDot=off  SenseRDot=off  SenseRotationSequenceDot=off  SenseAlphaX=off  SenseAlphaY=off  SenseAlphaZ=off  SenseQDDot=off  SenseRDDot=off  SenseX=off  SenseY=off  SenseZ=off  SenseRad=off  SenseAzim=off  SenseDist=off  SenseInc=off  SenseXDot=off  SenseYDot=off  SenseZDot=off  SenseRadDot=off  SenseAzimDot=off  SenseDistDot=off  SenseIncDot=off  SenseXDDot=off  SenseYDDot=off  SenseZDDot=off  SenseRadDDot=off  SenseAzimDDot=off  SenseDistDDot=off  SenseIncDDot=off
  vel2 sensor : sm_lib/Frames and Transforms/Transform Sensor  MeasurementFrame=World  RotationSequence=XYX  SenseAngle=on  SenseAxis=off  SenseQ=off  SenseR=off  SenseRotationSequence=off  SenseOmegaX=off  SenseOmegaY=off  SenseOmegaZ=on  SenseQDot=off  SenseRDot=off  SenseRotationSequenceDot=off  SenseAlphaX=off  SenseAlphaY=off  SenseAlphaZ=off  SenseQDDot=off  SenseRDDot=off  SenseX=off  SenseY=off  SenseZ=off  SenseRad=off  SenseAzim=off  SenseDist=off  SenseInc=off  SenseXDot=off  SenseYDot=off  SenseZDot=off  SenseRadDot=off  SenseAzimDot=off  SenseDistDot=off  SenseIncDot=off  SenseXDDot=off  SenseYDDot=off  SenseZDDot=off  SenseRadDDot=off  SenseAzimDDot=off  SenseDistDDot=off  SenseIncDDot=off
  X_end : Outport
  Y_end : Outport  Port=2
  Xd_end : Outport  Port=3
  Yd_end : Outport  Port=4
  Theta3 : Outport  Port=5
  q1 : Outport  Port=6
  q2 : Outport  Port=7
  q3 : Outport  Port=8
  q4 : Outport  Port=9
  qd1 : Outport  Port=10
  qd2 : Outport  Port=11
  qd3 : Outport  Port=12
  qd4 : Outport  Port=13
  wires:
  q1_desired/1 -> Simulink-PS Converter/1
  PS-Simulink Converter/1 -> q1/1
  PS-Simulink Converter4/1 -> q4/1
  q4_desired/1 -> Simulink-PS Converter3/1
  PS-Simulink Converter2/1 -> qd4/1
  PS-Simulink Converter1/1 -> qd1/1
  PS-Simulink Converter6/1 -> Y_end/1
  PS-Simulink Converter5/1 -> X_end/1
  PS-Simulink Converter8/1 -> Yd_end/1
  PS-Simulink Converter7/1 -> Xd_end/1
  PS-Simulink Converter10/1 -> qd2/1
  PS-Simulink Converter9/1 -> q2/1
  PS-Simulink Converter12/1 -> Theta3/1
  PS-Simulink Converter13/1 -> qd3/1
  PS-Simulink Converter14/1 -> q3/1
  connections:
  MechanismConfiguration/RConn1 -- pos3 sensor/LConn1 -- "Joint 3 sensor "/LConn1 -- vel2 sensor/LConn1 -- LBr vel sensor/LConn1 -- Solver Configuration/RConn1 -- Rigid Transform4/LConn1 -- Transform Sensor/LConn1 -- Rigid Transform5/LConn1 -- World/RConn1
  Transform Sensor/RConn1 -- Link Bl/RConn1 -- Joint P/LConn1
  Joint 3/LConn1 -- Link Br/LConn2
  Joint 1/RConn1 -- Rigid Transform/LConn1
  Rigid Transform/RConn1 -- Link Al/LConn1
  Link Ar/LConn1 -- Rigid Transform3/RConn1
  Joint 4/RConn1 -- Link Ar/LConn2
  Rigid Transform3/LConn1 -- Joint 3/RConn1
  Link Bl/LConn1 -- vel2 sensor/RConn1 -- Joint 2/RConn1
  Rigid Transform1/LConn1 -- Link Al/LConn2
  Joint P/RConn1 -- Rigid Transform2/LConn1
  Joint 4/RConn2 -- PS-Simulink Converter4/LConn1
  Simulink-PS Converter/RConn1 -- Joint 1/LConn2
  Joint 4/LConn2 -- Simulink-PS Converter3/RConn1
  PS-Simulink Converter/LConn1 -- Joint 1/RConn2
  Rigid Transform2/RConn1 -- Link Br/LConn1 -- Rigid Transform7/LConn1
  Joint 2/LConn1 -- Rigid Transform1/RConn1
  Joint 1/LConn1 -- Rigid Transform4/RConn1
  Transform Sensor/RConn2 -- PS-Simulink Converter5/LConn1
  PS-Simulink Converter6/LConn1 -- Transform Sensor/RConn3
  Rigid Transform5/RConn1 -- Joint 4/LConn1
  LBr vel sensor/RConn1 -- Rigid Transform6/RConn1
  Joint 1/RConn3 -- PS-Simulink Converter1/LConn1
  Joint 4/RConn3 -- PS-Simulink Converter2/LConn1
  LBr vel sensor/RConn2 -- PS-Simulink Converter7/LConn1
  LBr vel sensor/RConn3 -- PS-Simulink Converter8/LConn1
  PS-Simulink Converter9/LConn1 -- vel2 sensor/RConn2
  PS-Simulink Converter10/LConn1 -- vel2 sensor/RConn3
  pos3 sensor/RConn3 -- PS-Simulink Converter13/LConn1
  pos3 sensor/RConn2 -- PS-Simulink Converter14/LConn1
  pos3 sensor/RConn1 -- Rigid Transform8/LConn1 -- Rigid Transform7/RConn1 -- Rigid Transform6/LConn1
  "Joint 3 sensor "/RConn2 -- PS-Simulink Converter12/LConn1
  Rigid Transform8/RConn1 -- "Joint 3 sensor "/RConn1

== matlab function SCARA_Control_System/FK Function ==
  data: q1 input; x output; q4 input; y output
function [x, y] = forwardKinematics(q1, q4)
la = 0.100;
lb = 0.220;
lc = 0.230;

E = 2*lb*(lc + (la*(cos(q4) - cos(q1))));
F = (2*la*lb*sin(q4)) - (2*la*lb*sin(q1));
G = (lc^2) + (2*(la^2)) + (2*lc*la*cos(q4)) - (2*lc*la*cos(q1)) - (2*(la^2)*cos(q4 - q1));

theta2 = 2*atan((-F - sqrt( (E^2) + (F^2) - (G^2) )) / (G - E));

% display(theta2 * 180 / 3.1415);

x = lc + (la*cos(q4)) + (lb*cos(theta2));
y = (la*sin(q4)) + (lb*sin(theta2));

x = x - 0.115;

== matlab function SCARA_Control_System/IK Function ==
  data: Xp input; q1 output; Yp input; q4 output
function [q1, q4] = inverseKinematics(Xp, Yp)
%{ 
This function converts desired pose into angles of the actuated joints
@param Xp [1x1] -> Hor. distance in METERS from midpoint of motors line
@param Yp [1x1] -> Ver. distance in METERS from midpoint of motors line
return q1 [1x1] -> Angle in RAD of motor 1 (Left) from +ve x-axis CCW
return q2 [1x1] -> Angle in RAD of motor 2 (Right) from +ve x-axis CCW 
%}


la = 0.100; % Short link
lb = 0.220; % Long link
lc = 0.230; % Distance between motors

Xp = Xp + 0.115; % Mapping desired pose to motor 1 (Left | q1) axis

% -------------------------------------------------------------- 
% Pages(2-3) of [Baseline] reference file in "References" folder
% --------------------------------------------------------------

C = sqrt((Xp^2) + (Yp^2));
e = sqrt(((lc-Xp)^2) + (Yp^2));

q1 = atan(Yp/Xp) + acos((-(lb^2)+(la^2)+(C^2)) / (2*la*C));
q4 = 3.14 - atan((Yp)/(lc-Xp)) + acos((-(lb^2)+(la^2)+(e^2)) / (2*la*e));

== matlab function SCARA_Control_System/FJ Function ==
  data: q1 input; q4 input; Qd input; Xp input; Yp input; Xd output; Yd output
function [Xd, Yd] = forwardJacobian(q1, q4, Qd, Xp, Yp)
%{ 
This function converts joints velocities into endeffector velocity
@param Xp [1x1] -> Hor. distance in METERS from midpoint of motors line
@param Yp [1x1] -> Ver. distance in METERS from midpoint of motors line
@param q1 [1x1] -> Angle in RAD of motor 1 (Left) from +ve x-axis CCW
@param q4 [1x1] -> Angle in RAD of motor 2 (Right) from +ve x-axis CCW
@param Qd [4x1] -> Velocities in RAD/SEC of 4 joints (qd1,qd2,qd3,qd4)
return Xd -> Velocity in METER/SEC of the end-effector on x-axis
return Yd -> Velocity in METER/SEC of the end-effector on y-axis
%}

la = 0.100; % Sort link
lb = 0.220; % Long link
lc = 0.230; % Distance between motors

Xp = Xp + 0.115; % Mapping desired pose to motor 1 (Left | q1) axis

% ------------------------------------------------------------------
% Pages(7) Fig.2 of [Jacobian] reference file in "References" folder
% ------------------------------------------------------------------

r1 = 0; % Offset from end-effector along the long link (Right lb)
 
a1 = la;
a2 = lb;
a3 = lb;
a4 = la;

% Dependent joints
q2 = asin((Yp - (la*sin(q1))) / lb);
q3 = acos((Xp-lc-(la*cos(q4))) / lc);

% Jacobian matrix elements
J11 = -a1*sin(q1) + a1*(sin(q2)*sin(q3-q1)*a3 + r1*sin(q3)*sin(q1-q2))/a3/sin(q3-q2);
J12 = a4*(sin(q2)*sin(q4-q3)*a3 - r1*sin(q3)*sin(q4-q2))/a2/sin(q3-q2);
J21 = a1*cos(q1) - a1*(cos(q2)*sin(q3-q1)*a3 + r1*cos(q3)*sin(q1-q2))/a3/sin(q3-q2);
J22 = -a4*(cos(q2)*sin(q4-q3)*a3 - r1*cos(q3)*sin(q4-q2))/a3/sin(q3-q2);

% <<< NOTE >>> Eliminated part as angular speed aroud Z-axis not needed
%J31 = -a1*sin(q1-q2)/a3/sin(q3-q2);
%J32 = a4*sin(q4-q2)/a3/sin(q3-q2);

J = [J11 J12; J21 J22]; % Last row (J31 J32) in jacobian matrix not used 

V = J * [Qd(1); Qd(4)]; % End-effecor velocity matrix

Xd = V(1);
Yd = V(2);

== matlab function SCARA_Control_System/IJ Function ==
  data: q1 input; q4 input; Xd input; Xp input; Yp input; qd1 output; qd4 output
function [qd1, qd4] = inverseJacobian(q1, q4, Xd, Xp, Yp)
%{ 
This function converts desired endeffector velocity into joints velocities 
@param q1 [1x1] -> Angle in RAD of motor 1 (Left) from +ve x-axis CCW
@param q4 [1x1] -> Angle in RAD of motor 2 (Right) from +ve x-axis CCW
@param Xd [4x1] -> Velocities in METER/SEC of the end-effector
@param Xp [1x1] -> Hor. distance in METERS from midpoint of motors line
@param Yp [1x1] -> Ver. distance in METERS from midpoint of motors line

return qd1 -> Velocity in RAD/SEC of active joint 1 (Motor 1 | Left)
return qd4 -> Velocity in RAD/SEC of active joint 4 (Motor 2 | Right)
%}

la = 0.100; % Sort link
lb = 0.220; % Long link
lc = 0.230; % Distance between motors

Xp = Xp + 0.115; % Mapping desired pose to motor 1 (Left | q1) axis

% ------------------------------------------------------------------
% Pages(7) Fig.2 of [Jacobian] reference file in "References" folder
% ------------------------------------------------------------------

r1 = 0; % Offset from end-effector along the long link (Right lb)
 
a1 = la;
a2 = lb;
a3 = lb;
a4 = la;

% Dependent joints
q2 = asin((Yp - (la*sin(q1))) / lb);
q3 = acos((Xp-lc-(la*cos(q4))) / lc);

% Jacobian matrix elements
J11 = -a1*sin(q1) + a1*(sin(q2)*sin(q3-q1)*a3 + r1*sin(q3)*sin(q1-q2))/a3/sin(q3-q2);
J12 = a4*(sin(q2)*sin(q4-q3)*a3 - r1*sin(q3)*sin(q4-q2))/a2/sin(q3-q2);
J21 = a1*cos(q1) - a1*(cos(q2)*sin(q3-q1)*a3 + r1*cos(q3)*sin(q1-q2))/a3/sin(q3-q2);
J22 = -a4*(cos(q2)*sin(q4-q3)*a3 - r1*cos(q3)*sin(q4-q2))/a3/sin(q3-q2);

% <<< NOTE >>> Eliminated part as angular speed aroud Z-axis not needed
%J31 = -a1*sin(q1-q2)/a3/sin(q3-q2);
%J32 = a4*sin(q4-q2)/a3/sin(q3-q2);

J = [J11 J12; J21 J22]; % Last row (J31 J32) in jacobian matrix not used 

Qd = J \ [Xd(1); Xd(2)]; % Actuated Joints velocity matrix

qd1 = Qd(1);
qd4 = Qd(2);
